simulink model "TC"  (R2023b)
settings: Solver=VariableStepAuto  StartTime=0.0  StopTime=850  RelTol=1e-3
settings Model: Creator=joser  LastModifiedBy=joser

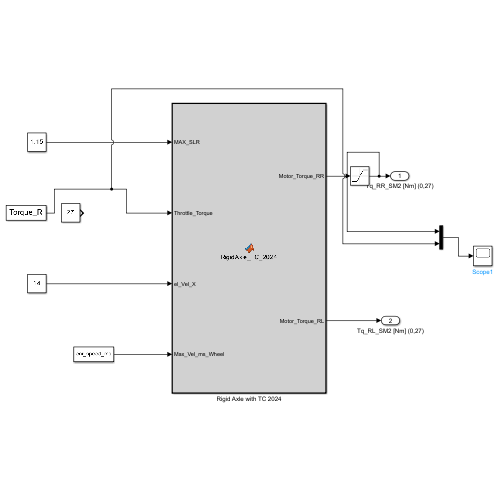
[thumbnail: Simulink's stored preview of the top-level diagram]
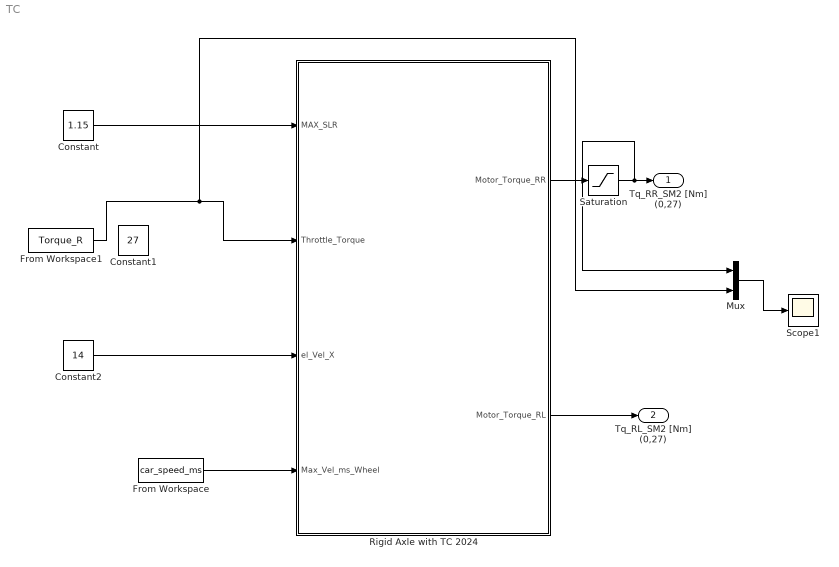
== system TC ==
  Constant : Constant  Value=1.15
  Constant1 : Constant  Value=27
  Constant2 : Constant  Value=14
  From Workspace : FromWorkspace  VariableName=car_speed_ms  SampleTime=0.005
  From Workspace1 : FromWorkspace  VariableName=Torque_R  SampleTime=0.005
  Mux : Mux  Inputs=2
  "Rigid Axle with TC 2024 " : MATLAB Function  TreatAsAtomicUnit=on
  Saturation : Saturate  UpperLimit=90  LowerLimit=0
  Scope1 : Scope
  Tq_RR_SM2 [Nm] (0,27) : Outport  VectorParamsAs1DForOutWhenUnconnected=off
  Tq_RL_SM2 [Nm] (0,27) : Outport  Port=2  VectorParamsAs1DForOutWhenUnconnected=off
  wires:
  Constant/1 -> "Rigid Axle with TC 2024 "/1(MAX_SLR)
  Constant2/1 -> "Rigid Axle with TC 2024 "/3(el_Vel_X)
  From Workspace/1 -> "Rigid Axle with TC 2024 "/4(Max_Vel_ms_Wheel)
  "Rigid Axle with TC 2024 "/2(Motor_Torque_RL) -> Tq_RL_SM2 [Nm] (0,27)/1
  From Workspace1/1 -> Mux/2, "Rigid Axle with TC 2024 "/2(Throttle_Torque)
  Mux/1 -> Scope1/1
  "Rigid Axle with TC 2024 "/1(Motor_Torque_RR) -> Saturation/1
  Saturation/1 -> Mux/1, Tq_RR_SM2 [Nm] (0,27)/1

== matlab function TC/Rigid Axle with TC 2024  ==
  data: MAX_SLR input; Throttle_Torque input; Motor_Torque_RR output; Motor_Torque_RL output; el_Vel_X input; Max_Vel_ms_Wheel input
function [Motor_Torque_RR, Motor_Torque_RL] = RigidAxle_TC_2024(MAX_SLR, Throttle_Torque, el_Vel_X, Max_Vel_ms_Wheel)    
    persistent correction
    if isempty(correction)
        correction = 0;
    end
if (el_Vel_X < 0.5 || Max_Vel_ms_Wheel < 0.5)
    correction = 0;
    Motor_Torque_RR = Throttle_Torque;
    Motor_Torque_RL = Throttle_Torque;
    return;
else

% SLIP RATIO CALCULATIONS
    % calculate slip ratio
    if(el_Vel_X == 0 ||Max_Vel_ms_Wheel == 0)
        SLR = 1;
    else
    SLR = (Max_Vel_ms_Wheel / el_Vel_X);
    end
% CHECK FOR EXCESIVE SLIPPING
    % SLIP RATIO LESSER THAN MAXIMUM SLIP RATIO => apply max torque times throttle factor
        if(SLR < MAX_SLR)
            Motor_Torque_RR = Throttle_Torque; 
            Motor_Torque_RL = Throttle_Torque;
            correction = 0; %set correction to 0 as tyre is not slipping
            return;
        else
        % TYRE SLIPPING => TC INTERVENES
            % LOOK FOR THE PREVIOUS CORRECTION [Nm]
            if (correction == 0) % NOT SLIPPING PREVIOUSLY
                correction = 1; % [INTERVAL TO BE DETERMINED] set the correction to the torque we want to substract
                Motor_Torque_RR = Throttle_Torque - (1/33*correction^2+1/33*correction); % substract the correction from the torque to apply
                Motor_Torque_RL = Throttle_Torque - (1/33*correction^2+1/33*correction);
                return;
            else % TYRE SLIPPING PREVIOUSLY
                correction = correction + 1; % [INTERVAL TO BE DETERMINED] set the correction to the torque we want to substract + previous corrections
                Motor_Torque_RR = Throttle_Torque - (1/33*correction^2+1/33*correction); % substract the correction from the torque to apply
                Motor_Torque_RL = Throttle_Torque - (1/33*correction^2+1/33*correction);
                return;
            end
        end
end
end
